simulink model "requriment_333"  (R2021a)
settings: Solver=FixedStepDiscrete  StartTime=0.0  StopTime=50  FixedStep=1  RelTol=1e-3
libraries: simulink x3
settings Model: Creator=Rahul  LastModifiedBy=Rahul
settings ConfigComp: CovMetricSettings=dcmwe

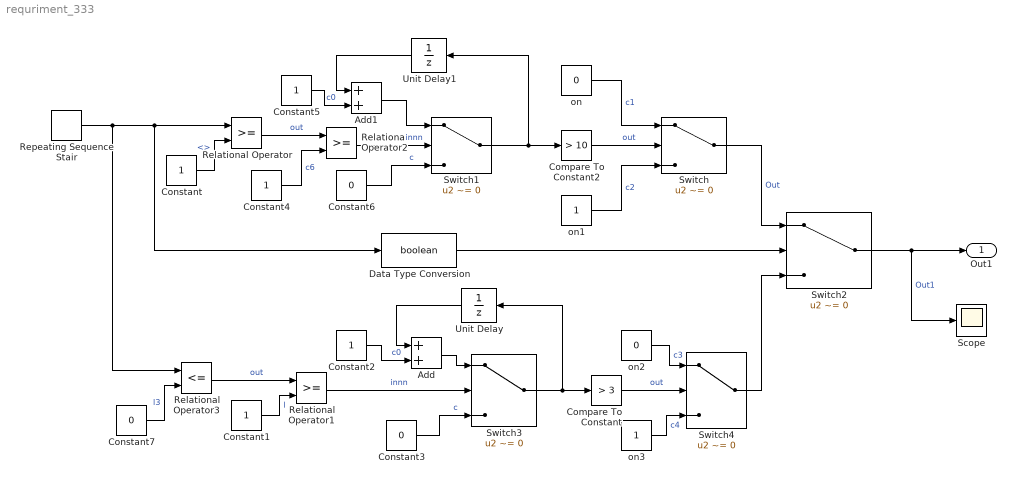
== system requriment_333 ==
  Add : Sum
  Add1 : Sum
  Compare To Constant : simulink/Logic and Bit Operations/Compare To Constant  relop=>  const=3  OutDataTypeStr=boolean
  Compare To Constant2 : simulink/Logic and Bit Operations/Compare To Constant  relop=>  const=10  OutDataTypeStr=boolean
  Constant{,1..2,4..5} (5 alike) : Constant
  Constant3 : Constant  Value=0
  Constant6 : Constant  Value=0
  Constant7 : Constant  Value=0
  Data Type Conversion : DataTypeConversion  OutDataTypeStr=boolean
  Relational Operator : RelationalOperator  OutDataTypeStr=boolean  RndMeth=Simplest
  Relational Operator1 : RelationalOperator  OutDataTypeStr=boolean  RndMeth=Simplest
  Relational Operator2 : RelationalOperator  OutDataTypeStr=boolean  RndMeth=Simplest
  Relational Operator3 : RelationalOperator  Operator=<=  OutDataTypeStr=boolean  RndMeth=Simplest
  Repeating Sequence Stair : simulink/Sources/Repeating Sequence Stair  OutValues=[1 1 1 1 1 1 1 1 1 1 1 0 0 0 0 0]  tsamp=-1  OutMin=[]  OutMax=[]  OutDataTypeStr=double  OutputDataTypeScalingMode=double  OutDataType=fixdt(0,8)  ConRadixGroup=Best Precision: Vector-wise  OutScaling=2^-12
  Scope : Scope
  Switch : Switch  Criteria=u2 ~= 0  OutDataTypeStr=boolean
  Switch1 : Switch  Criteria=u2 ~= 0
  Switch2 : Switch  Criteria=u2 ~= 0  OutDataTypeStr=boolean
  Switch3 : Switch  Criteria=u2 ~= 0
  Switch4 : Switch  Criteria=u2 ~= 0
  Unit Delay : UnitDelay  SampleTime=-1  HasFrameUpgradeWarning=on
  Unit Delay1 : UnitDelay  SampleTime=-1  HasFrameUpgradeWarning=on
  on : Constant  Value=0  OutDataTypeStr=boolean
  on1 : Constant
  on2 : Constant  Value=0  OutDataTypeStr=boolean
  on3 : Constant
  Out1 : Outport  VectorParamsAs1DForOutWhenUnconnected=off
  wires:
  Relational Operator/1 -> Relational Operator2/1  "out"
  Constant/1 -> Relational Operator/2  "<>"
  Constant5/1 -> Add1/2  "c0"
  Switch1/1 -> Unit Delay1/1, Compare To Constant2/1
  Add1/1 -> Switch1/1
  Unit Delay1/1 -> Add1/1
  Constant4/1 -> Relational Operator2/2  "c6"
  Constant6/1 -> Switch1/3  "c"
  Compare To Constant2/1 -> Switch/2  "out"
  Relational Operator2/1 -> Switch1/2  "innn"
  on/1 -> Switch/1  "c1"
  on1/1 -> Switch/3  "c2"
  Switch/1 -> Switch2/1  "Out"
  Switch2/1 -> Scope/1, Out1/1  "Out1"
  Data Type Conversion/1 -> Switch2/2
  Switch4/1 -> Switch2/3
  Constant2/1 -> Add/2  "c0"
  Repeating Sequence Stair/1 -> Relational Operator3/1, Data Type Conversion/1, Relational Operator/1
  Constant3/1 -> Switch3/3  "c"
  Relational Operator1/1 -> Switch3/2  "innn"
  Constant1/1 -> Relational Operator1/2  "l"
  Compare To Constant/1 -> Switch4/2  "out"
  Unit Delay/1 -> Add/1
  Switch3/1 -> Unit Delay/1, Compare To Constant/1
  Add/1 -> Switch3/1
  on3/1 -> Switch4/3  "c4"
  on2/1 -> Switch4/1  "c3"
  Constant7/1 -> Relational Operator3/2  "l3"
  Relational Operator3/1 -> Relational Operator1/1  "out"
